simulink model "modelo"  (R2020b)
settings: Solver=VariableStepAuto  StartTime=0.0  StopTime=10.0  RelTol=1e-3
values from neighbouring files (symbols this model uses):
  E = 100    [ejercicio7.m]
  f = 50    [ejercicio7.m]
  L = 50e-3    (= 0.05)    [ejercicio7.m]
  R = 10    [ejercicio7.m]
libraries: powerlib x4
settings Model: Creator=Aitor  LastModifiedBy=Aitor

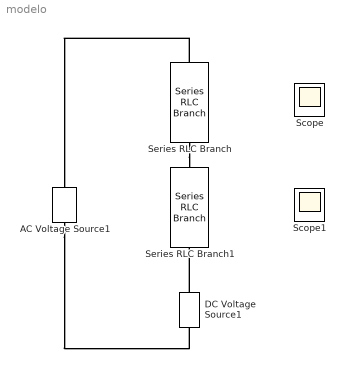
== system modelo ==
  AC Voltage Source1 : powerlib/Electrical Sources/AC Voltage Source  Amplitude=1  Phase=0  Frequency=f  SampleTime=0  Measurements=None  BusType=swing  Pref=10e3  Qref=0  Qmin=-inf  Qmax=+inf
  DC Voltage Source1 : powerlib/Electrical Sources/DC Voltage Source  Amplitude=E  Measurements=None
  Scope : Scope  NumInputPorts=2
  Scope1 : Scope  NumInputPorts=2
  Series RLC Branch : powerlib/Elements/Series RLC Branch  LConnTagsString=__new0  RConnTagsString=__new0  BranchType=R  Resistance=R  Inductance=1e-3  SetiL0=off  InitialCurrent=0  Capacitance=1e-6  Setx0=off  InitialVoltage=0  Measurements=None
  Series RLC Branch1 : powerlib/Elements/Series RLC Branch  LConnTagsString=__new0  RConnTagsString=__new0  BranchType=L  Resistance=1  Inductance=L  SetiL0=off  InitialCurrent=0  Capacitance=1e-6  Setx0=off  InitialVoltage=0  Measurements=None
  connections:
  Series RLC Branch/RConn1 -- Series RLC Branch1/LConn1
  Series RLC Branch/LConn1 -- AC Voltage Source1/RConn1
  DC Voltage Source1/RConn1 -- Series RLC Branch1/RConn1
  AC Voltage Source1/LConn1 -- DC Voltage Source1/LConn1
